simulink model "Airfield_a"  (R2021a)
settings: Solver=VariableStepAuto  StartTime=0.0  StopTime=10.0  RelTol=1e-3
libraries: aerolibconvert2 x2, simulink x1
settings Model: Creator=Charis  LastModifiedBy=wardb

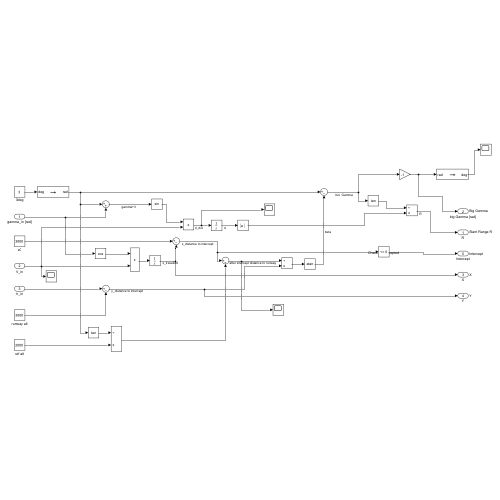
[thumbnail: Simulink's stored preview of the top-level diagram]
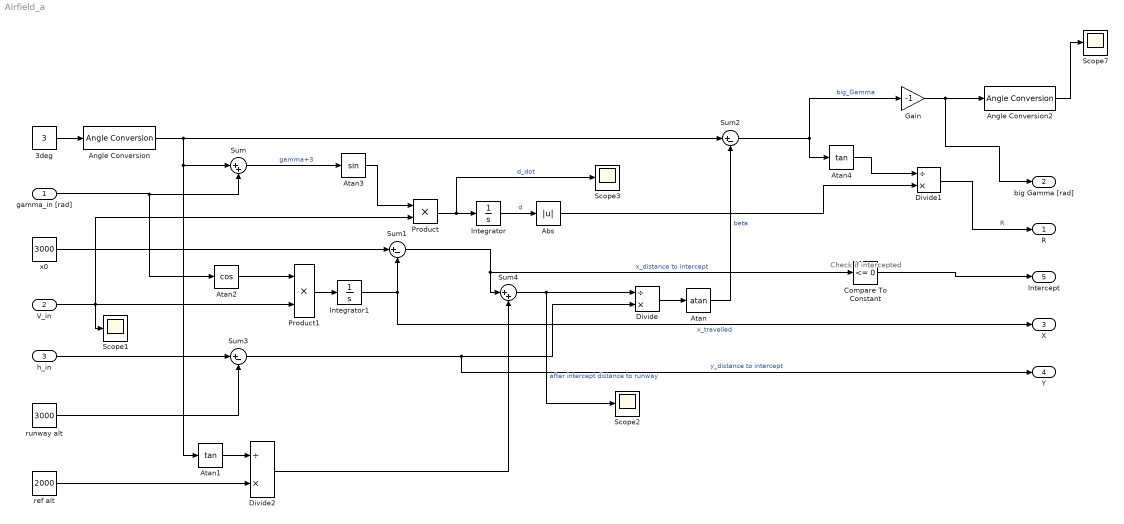
== system Airfield_a ==
  note: Check if intercepted
  gamma_in [rad] : Inport
  V_in : Inport  Port=2
  h_in : Inport  Port=3
  3deg : Constant  Value=3
  Abs : Abs
  Angle Conversion : aerolibconvert2/Angle Conversion  IU=deg  OU=rad
  Angle Conversion2 : aerolibconvert2/Angle Conversion  IU=rad  OU=deg
  Atan : Trigonometry  Operator=atan
  Atan1 : Trigonometry  Operator=tan
  Atan2 : Trigonometry  Operator=cos
  Atan3 : Trigonometry
  Atan4 : Trigonometry  Operator=tan
  Compare To Constant : simulink/Logic and Bit Operations/Compare To Constant  relop=<=  const=0  OutDataTypeStr=boolean
  Divide : Product  Inputs=/*
  Divide1 : Product  Inputs=/*
  Divide2 : Product  Inputs=/*
  Gain : Gain  Gain=-1
  Integrator : Integrator
  Integrator1 : Integrator
  Product : Product
  Product1 : Product
  Scope{1..3,7} (4 alike) : Scope
  Sum : Sum  Inputs=|++
  Sum1 : Sum  Inputs=|+-
  Sum2 : Sum  Inputs=|+-
  Sum3 : Sum  Inputs=|+-
  Sum4 : Sum  Inputs=|++
  ref alt : Constant  Value=2000
  runway alt : Constant  Value=3000
  x0 : Constant  Value=3000
  R : Outport  SignalName=Slant Range R
  big Gamma [rad] : Outport  Port=2  SignalName=Big Gamma
  X : Outport  Port=3  SignalName=X
  Y : Outport  Port=4  SignalName=Y
  Intercept : Outport  Port=5  SignalName=Intercept
  wires:
  Sum/1 -> Atan3/1  "gamma+3"
  Product/1 -> Scope3/1, Integrator/1  "d_dot"
  V_in/1 -> Product1/2, Product/2, Scope1/1
  Atan2/1 -> Product1/1
  Product1/1 -> Integrator1/1
  h_in/1 -> Sum3/1
  Sum1/1 -> Compare To Constant/1, Sum4/1  "x_distance to intercept"
  Divide/1 -> Atan/1
  Atan/1 -> Sum2/2  "beta"
  Sum2/1 -> Atan4/1, Gain/1  "big_Gamma"
  Divide1/1 -> R/1  "R"
  3deg/1 -> Angle Conversion/1
  Atan3/1 -> Product/1
  runway alt/1 -> Sum3/2
  Sum3/1 -> Y/1, Divide/2  "y_distance to intercept"
  Compare To Constant/1 -> Intercept/1
  ref alt/1 -> Divide2/2
  Atan1/1 -> Divide2/1
  Divide2/1 -> Sum4/2
  Sum4/1 -> Scope2/1, Divide/1  "after intercept distance to runway"
  Angle Conversion2/1 -> Scope7/1
  Gain/1 -> big Gamma [rad]/1, Angle Conversion2/1
  Integrator1/1 -> Sum1/2, X/1  "x_travelled"
  x0/1 -> Sum1/1
  Atan4/1 -> Divide1/1
  Integrator/1 -> Abs/1  "d"
  Abs/1 -> Divide1/2
  Angle Conversion/1 -> Atan1/1, Sum/1, Sum2/1
  gamma_in [rad]/1 -> Atan2/1, Sum/2
